simulink model "AutonomousScan"  (R2019a)
settings: Solver=FixedStepAuto  StartTime=0.0  StopTime=inf  FixedStep=0.001  RelTol=1e-3
libraries: dspnetwork x24, simulink_extras x3, etargetslib x1, dspmtrx3 x1, dspstat3 x1, simulink x1
(part 2 of 2)

== matlab function AutonomousScan/Trajectory Generation1 ==
  settings: updateMethod=DISCRETE
  data: pos_des output; current_pos input; record_data output; measured_force input; bias_good input
function [pos_des, record_data] = fcn( current_pos, measured_force, bias_good)
persistent k contact_made pnt 

if isempty(k)
    k = 1;
end

if isempty(contact_made)
    contact_made = false;
end

if isempty(pnt)
    pnt = 1;
end

%constants
trajectory = [0.45 0 0;
    0.475 -0.025 0;
    0.425 -0.025 0;
    0.415 0 0;
    0.485 0 0;
    0.475 0.025 0;
    0.425 0.025 0
    0.425 0.025 0];
pos_max_error = 0.0007;
pos_max_error_fine = 0.00005;
contact_force = -1.1;
smooth_traj = repmat(trajectory(1,:), 8000, 1);

%set contact flag by measuring z force
if bias_good == true && measured_force(3) <= contact_force
    contact_made = true;
end

%selective recording
if contact_made == true && mod(k,2) == 0
    record_data = 1;
else
    record_data = 0;
end

%generates vector between current and next point
vect = trajectory(k+1,:) - trajectory(k,:);

%generates trajectory between adjecent points
if contact_made == true
    for t = 1:5000
        smooth_traj(t,:) = trajectory(k,:) + (t/5000).*vect;
    end
    
    %SEND MORE OF FINAL POINT
    v = smooth_traj(5000,:);
    smooth_traj = [smooth_traj(1:5000,:); repmat(v,3000,1)];
    
    %SEND MORE OF EACH POINT
    %smooth_traj = repelem(smooth_traj(1:40,:), 1000, 1);
end

%send desired coordinates to robot
pos_des = smooth_traj(pnt, :).';

%checks if vector end point has been reached
err_pos = sum(abs(current_pos(1:2,1) - trajectory(k+1,1:2).'));
if contact_made == true && err_pos <= pos_max_error
    
    %switches to next set of adjacent points
    k = k + 1;
    
    %checks if end of trajectory
    if k == size(trajectory, 1)
        k = 7;
    end
    
    %reset counter
    pnt = 1;
end

if contact_made == true
    pnt = pnt + 1;
    if pnt == 8001
        pnt = 1;
    end
end

end


% %WAIT UNTIL REACHES EACH POINT
% err_pos_fine = sum(abs(current_pos(1:2,1) - desired_pos(1:2,1)));
% 
% pos_des = smooth_traj(pnt, :).';
% 
% if contact_made == true && err_pos_fine <= pos_max_error_fine
%     pnt = pnt +1;
%     if pnt == 8
%         pnt = 1;
%     end
% end

== matlab function AutonomousScan/MATLAB Function9 ==
  data: u input; V_cart_2 output; panda_pos input
function V_cart_2 = fcn(u, panda_pos)
persistent n
if isempty(n)
    n=1;
end

desPos = u(1:2,1)/100;

V_cart_2 = [desPos - panda_pos(1:2);0];

== matlab function AutonomousScan/MATLAB Function10 ==
  data: sensor input; y output
function y = fcn(sensor)
persistent n origSensor

if isempty(n)
    n = 1;
end

if isempty(origSensor)
    origSensor = zeros(7,1);
end

if n == 1 && sensor(1)~=0
    origSensor = sensor;
    
    n = 2;
end    

y = origSensor;

== matlab function AutonomousScan/MATLAB Function11 ==
  data: panda_pos input; y output; intraop input
function y = fcn(panda_pos, intraop)
persistent n origPanda

if isempty(n)
    n = 1;
end

if isempty(origPanda)
    origPanda = zeros(3,1);
end

if n == 1 && panda_pos(1)~=0 && intraop == 1
    origPanda = panda_pos;
    
    n = 2;
end    

y = origPanda;

== matlab function AutonomousScan/MATLAB Function12 ==
  data: y output; limit output
function [y, limit] = fcn()
persistent n

if isempty(n)
    n = 0;
end

n=n+1;

if n<=5000
    y = [0 0 0 0 0 0 0];
elseif n>5000 && n<= 10000
    y = [0 0 0 0 1 0 0];
elseif n>10000 && n<=15000
    y = [0 0 0 0 0 0 0];
else
    y = [0 0 0 0 1 0 0];
end


limit = n;

== matlab function AutonomousScan/MATLAB Function13 ==
  data: u input; y output
function y = fcn(u)
    for i = 1:3
        if u(i)>pi
            u(i) = u(i)-(2*pi)
        elseif u(i)<-pi
            u(i) = u(i)+(2*pi)
        end
    end
y = u;

== matlab function AutonomousScan/MATLAB Function14 ==
  data: rcm input; rotmat output; tip input; currentZ input
function rotmat = fcn(rcm, tip, currentZ)

newZ = tip-rcm;
newZ = newZ/norm(newZ);
normPlane = cross(currentZ, newZ);

axisRot = normPlane/norm(normPlane);
nx = axisRot(1);
ny = axisRot(2);
nz = axisRot(3);

theta = acos(dot(currentZ,newZ)/(norm(currentZ)*norm(newZ)));

v=1-cos(theta);
c=cos(theta);
s=sin(theta);

rotmat =[nx^2*v+c,nx*ny*v-nz*s,nx*nz*v+ny*s;...
                              nx*ny*v+nz*s,ny^2*v+c,ny*nz*v-nx*s;
                              nx*nz*v-ny*s,ny*nz*v+nx*s,nz^2*v+c];

== matlab function AutonomousScan/in general3 ==
  data: grad output; brad output; arad output; R input
function [grad,brad,arad] = so3_to_rpy(R)
sy = sqrt(R(3,2)^2 + R(3,3)^2);
if sy > eps
    % non singular
    grad = atan2(R(3,2),R(3,3));
    brad = atan2(-R(3,1),sy);
    arad = atan2(R(2,1),R(1,1));
else
    % singular
    grad = atan2(-R(2,3),R(2,2));
    brad = atan2(-R(3,1),sy);
    arad = 0;
end
end

== matlab function AutonomousScan/MATLAB Function15 ==
  data: R output; arad input; brad input; grad input
function R  = rot(arad,brad,grad)
%#codegen
Rz = [cos(arad) -sin(arad) 0; sin(arad) cos(arad) 0; 0 0 1];
Ry = [cos(brad) 0 sin(brad); 0 1 0; -sin(brad) 0 cos(brad)];
Rx = [1 0 0; 0 cos(grad) -sin(grad); 0 sin(grad) cos(grad)];
R = Rz * Ry * Rx;

== matlab function AutonomousScan/MATLAB Function16 ==
  data: R output; arad input; brad input; grad input
function R  = rot(arad,brad,grad)
%#codegen
Rz = [cos(arad) -sin(arad) 0; sin(arad) cos(arad) 0; 0 0 1];
Ry = [cos(brad) 0 sin(brad); 0 1 0; -sin(brad) 0 cos(brad)];
Rx = [1 0 0; 0 cos(grad) -sin(grad); 0 sin(grad) cos(grad)];
R = Rz * Ry * Rx;

== matlab function AutonomousScan/MATLAB Function18 ==
  data: R output; arad input; brad input; grad input
function R  = rot(arad,brad,grad)
%#codegen
Rz = [cos(arad) -sin(arad) 0; sin(arad) cos(arad) 0; 0 0 1];
Ry = [cos(brad) 0 sin(brad); 0 1 0; -sin(brad) 0 cos(brad)];
Rx = [1 0 0; 0 cos(grad) -sin(grad); 0 sin(grad) cos(grad)];
R = Rz * Ry * Rx;

== matlab function AutonomousScan/in general4 ==
  data: grad output; brad output; arad output; R input
function [grad,brad,arad] = so3_to_rpy(R)
sy = sqrt(R(3,2)^2 + R(3,3)^2);
if sy > eps
    % non singular
    grad = atan2(R(3,2),R(3,3));
    brad = atan2(-R(3,1),sy);
    arad = atan2(R(2,1),R(1,1));
else
    % singular
    grad = atan2(-R(2,3),R(2,2));
    brad = atan2(-R(3,1),sy);
    arad = 0;
end
end

== matlab function AutonomousScan/MATLAB Function20 ==
  data: u input; y output
function y = fcn(u)
    for i = 1:3
        if u(i)>pi
            u(i) = u(i)-(2*pi)
        elseif u(i)<-pi
            u(i) = u(i)+(2*pi)
        end
    end
y = u;

== matlab function AutonomousScan/MATLAB Function21 ==
  data: R input; T output; P input
function T = fcn(R, P)

T = [R P; 0 0 0 1];

== matlab function AutonomousScan/MATLAB Function22 ==
  data: u input; y output
function y = fcn(u)
y = u(1:3,end);

== matlab function AutonomousScan/MATLAB Function23 ==
  data: u input; y output
function y = fcn(u)
y=inv(u);

== matlab function AutonomousScan/MATLAB Function24 ==
  data: u input; y output
function y = fcn(u)
y=inv(u);

== matlab function AutonomousScan/MATLAB Function25 ==
  data: u input; y output
function y = fcn(u)
y = u(1:3,end);

== matlab function AutonomousScan/MATLAB Function26 ==
  data: pandaDes output; sensor input; quat output; sensorCurrent output; pandaCurrent input; rotZ input
function [pandaDes, quat, sensorCurrent]  = fcn(sensor, pandaCurrent, rotZ)
persistent transform transform2

if isempty(transform)
%     transform = [
%     0.0157   -0.0208   -0.9820   -0.0000
%     1.0071    0.0053    0.0197    0.0000
%     0.0034   -1.0071    0.0285   -0.0000
%     0.4598   -0.2811    0.0175    1.0000];

transform = [
    0.1742    0.9918    0.5463    0.0000
    0.8595   -0.7297   -0.0298    0.0000
   -0.1544   -0.9591   -0.0756   -0.0000
    0.3959   -0.3642    0.3008    1.0000
];
end


if isempty(transform2)
    transform2 = [
    0.0157   -0.0208   -0.9820   -0.0000
    1.0071    0.0053    0.0197    0.0000
    0.0034   -1.0071    0.0285   -0.0000
    0.4598   -0.2811    0.0175    1.0000];

end

sensorPos = [sensor(1:3)'./1000 1];
pandaPos = sensorPos * transform;
sensorCurrent = sensorPos*transform2;

% pandaPos(1) = pandaPos(1) - 0.2*sin(rotZ) + 0.0036;
% pandaPos(2) = pandaPos(2) - 0.2*cos(rotZ) - 0.0092;
%pandaPos(1) = sensorCurrent(1)-(abs(pandaPos(1)-sensorCurrent(1)))*sin(rotZ);
%pandaPos(2) = sensorCurrent(2)-(abs(pandaPos(2)-sensorCurrent(2)))*cos(rotZ);


if abs(sensorPos(1)) > 1000 || abs(sensorPos(2)) > 1000 || abs(sensorPos(3)) > 1000
    pandaPos = [pandaCurrent(1) pandaCurrent(2) pandaCurrent(3) 1];
end

pandaDes = [pandaPos(1:2) 0]';


quat = sensor(4:7);

== matlab function AutonomousScan/MATLAB Function27 ==
  data: u input; y output
function y = fcn(u)
    for i = 1:3
        if u(i)>pi
            u(i) = u(i)-(2*pi)
        elseif u(i)<-pi
            u(i) = u(i)+(2*pi)
        end
    end
y = u;

== matlab function AutonomousScan/Trajectory Generation (works) ==
  settings: updateMethod=DISCRETE
  data: shutter_fb input; pos_des output; current_pos input; record_data output; measured_force input; bias_good input; shutter output; pnts output; scan_complete output
function [pos_des, record_data, shutter, pnts, scan_complete] = fcn(shutter_fb, current_pos, measured_force, bias_good)
persistent k contact_made pnt shutter_pass

if isempty(k)
    k = 1;
end

if isempty(contact_made)
    contact_made = false;
end

if isempty(pnt)
    pnt = 1;
end

if isempty(shutter_pass)
    shutter_pass = 0;
end

%change to 0 when need to scan
scan_complete = 1;

%constants
trajectory = [0.45 0 0;
    0.475 -0.025 0;
    0.425 -0.025 0;
    0.415 0 0;
    0.485 0 0;
    0.475 0.025 0;
    0.425 0.025 0
    0.425 0.025 0];
pos_max_error_fine = 0.0001;
x_dist = 0.00125; %(0.475-0.425)/25
contact_force = -1.1;
% num_points = ceil(abs(trajectory(k+1,1)-trajectory(k,1))/x_dist);
num_points = ceil(abs(max(trajectory(:,1))-min(trajectory(:,1)))/x_dist)+1;

smooth_traj = repmat(trajectory(1,:), num_points, 1); 
shutter = 0;

%set contact flag by measuring z force
if bias_good == true && measured_force(3) <= contact_force
    contact_made = true;
end

%selective recording
% if contact_made == true && mod(k,2) == 0
if mod(k,2) == 0
    record_data = 1;
else
    record_data = 0;
end

%generates trajectory between adjecent points
if record_data == 1
    if trajectory(k,1) > trajectory(k+1,1)
        x_dist = -x_dist;
    end
        
    for t = 1:num_points
        smooth_traj(t,:) = [trajectory(k,1)+(t-1)*x_dist trajectory(k,2) trajectory(k,3)]; 
    end

elseif contact_made == true && record_data == 0 
    for t = 1:num_points
        smooth_traj(t,:) = trajectory(k+1,:);
    end
end

%send desired coordinates to robot
pos_des = smooth_traj(pnt, :).';

err_pos_fine = sum(abs(current_pos(1:2,1) - pos_des(1:2,1)));
if record_data == 1 && err_pos_fine <= pos_max_error_fine

    shutter_pass = 1; 
    
    if shutter_fb == 1
        pnt = pnt + 1;
        if pnt > num_points
            pnt = 1;
        end
        shutter_pass = 0;
    end
end

%checks if vector end point has been reached
err_pos = sum(abs(current_pos(1:2,1) - trajectory(k+1,1:2).'));
if contact_made == true && err_pos <= pos_max_error_fine
    
    shutter_pass = 1;
    
    if shutter_fb == 1
        %switches to next set of adjacent points
        k = k + 1;
        
        %checks if end of trajectory
        if k == size(trajectory, 1)
            k = size(trajectory, 1) - 1;
        end
        scan_complete = 1;
        %reset counter
        pnt = 1;
        shutter_pass = 0;
    end
    
    if k == size(trajectory, 1) - 1
        shutter_pass = 0;
    end
end

if shutter_pass == 1 && shutter_fb ~= 1
    shutter = 1;
end



pnts = pnt;
end

== matlab function AutonomousScan/MATLAB Function28 ==
  data: pandaPos input; pandaDes output
function pandaDes   = safetybox(pandaPos)
safetyboxX = [0.1 0.55];
safetyboxY = [-0.25 0.18];

if pandaPos(1) < safetyboxX(1)
    pandaPos(1) = safetyboxX(1);
elseif pandaPos(1) > safetyboxX(2)
    pandaPos(1) = safetyboxX(2);
end

if pandaPos(2) < safetyboxY(1)
    pandaPos(2) = safetyboxY(1);
elseif pandaPos(2) > safetyboxY(2)
    pandaPos(2) = safetyboxY(2);
end

pandaDes = [pandaPos(1:2); 0];

== matlab function AutonomousScan/MATLAB Function29 ==
  data: motoman_transform output; message input; hole output
function [motoman_transform, hole] = transform(message)

motoman_transform = [message(4:6)' ,message(1); message(7:9)', message(2); message(10:12)', message(3); 0 0 0 1];

current_motoman = [
    0.07043 0.9957 -0.06055 0.4181; 
    -0.02056 0.06214 0.9979 -0.06345; 
    0.9973 -0.06903 0.02485 0.2356]; 

newrotm = motoman_transform(1:3,1:3)*current_motoman(1:3,1:3); 

%motoman_offset = [1 0 0 (0.08352*sin(message(15)+2.8798)); 0 1 0 (0.08352*cos(message(15)+2.8798)); 0 0 1 -0.03; 0 0 0 1];
motoman_offset = [1 0 0 0.08352; 0 1 0 0.0108; 0 0 1 -0.03; 0 0 0 1];

desired_pos = newrotm*motoman_offset(1:3,4) + current_motoman(1:3,4);

transform = [
    0.0004   -0.9408    0.0079    0.0000
    0.9961    0.0739    0.0126   -0.0000
    0.0018   -0.0364    1.0297   -0.0000
    0.4523    0.5418   -0.1090    1.0000
];

tf = transform'*[motoman_transform(1:3,1:3) desired_pos; 0 0 0 1]; 
%tf = transform' *motoman_offset * motoman_transform  ; 

hole = tf(1:3,4);
end

== matlab function AutonomousScan/in general1 ==
  data: grad output; brad output; arad output; R input
function [grad,brad,arad] = so3_to_rpy(R)
sy = sqrt(R(3,2)^2 + R(3,3)^2);
if sy > eps
    % non singular
    grad = atan2(R(3,2),R(3,3));
    brad = atan2(-R(3,1),sy);
    arad = atan2(R(2,1),R(1,1));
else
    % singular
    grad = atan2(-R(2,3),R(2,2));
    brad = atan2(-R(3,1),sy);
    arad = 0;
end
end

== matlab function AutonomousScan/MATLAB Function30 ==
  data: rotZ output; input input
function rotZ   = filter(input)
persistent rotZ_dummy

if isempty(rotZ_dummy)
    rotZ_dummy = 0;
end 

if input > 4
    rotZ = rotZ_dummy;
else
    rotZ_dummy = input;
    rotZ = input;
end  
    

end

== matlab function AutonomousScan/MATLAB Function31 ==
  data: needletip_pos output; hole input; sensor input; needle output; unitneedle output
function [needletip_pos, needle, unitneedle]  = offset(hole, sensor)
persistent needletip_dummy

if isempty(needletip_dummy)
    needletip_dummy = [0.5 0 0];
end 

needle = [(hole(1) - sensor(1)) (hole(2) - sensor(2)) 0]; 

unitneedle = needle/norm(needle);  

needletip_test = [(sensor(1) + 0.2*unitneedle(1)) (sensor(2) + 0.2*unitneedle(2)) 0];

if abs(needletip_test(1)) > 1000 || abs(needletip_test(2)) > 1000
    needletip_pos = needletip_dummy;
else
    needletip_dummy = needletip_test;
    needletip_pos = needletip_test;
end  
    

end

== matlab function AutonomousScan/MATLAB Function32 ==
  data: motoman_transform output; message input; needletip_pos output; sensor input; motoman_pos output; motoman_rpy output
function [motoman_transform, needletip_pos, motoman_pos, motoman_rpy]  = transform(message, sensor)
persistent needletip_dummy

if isempty(needletip_dummy)
    needletip_dummy = [0.5 0 0];
end 

motoman_transform = [message(4:6)' ,message(1); message(7:9)', message(2); message(10:12)', message(3); 0 0 0 1];
%current_motoman = [0.0153 0.0582 0.9982 0.4147; -0.0478 -0.9971 0.0589 0.0060; 0.9987 -0.0486 -0.0125 0.2397]; 
%newrotm = motoman_transform(1:3,1:3)*current_motoman(1:3,1:3); 
%motoman_offset = [1 0 0 (0.08352*sin(message(15)+2.8798)); 0 1 0 (0.08352*cos(message(15)+2.8798)); 0 0 1 -0.03; 0 0 0 1];
%motoman_offset = [1 0 0 0.08352; 0 1 0 0.0108; 0 0 1 -0.03; 0 0 0 1];

current_motoman = [
    0.07043 0.9957 -0.06055 0.4181; 
    -0.02056 0.06214 0.9979 -0.06345; 
    0.9973 -0.06903 0.02485 0.2356]; 

transform_sensor = [
    0.0157   -0.0208   -0.9820   -0.0000
    1.0071    0.0053    0.0197    0.0000
    0.0034   -1.0071    0.0285   -0.0000
    0.4598   -0.2811    0.0175    1.0000];

transform_motoman = [    
    0.0004   -0.9408    0.0079    0.0000
    0.9961    0.0739    0.0126   -0.0000
    0.0018   -0.0364    1.0297   -0.0000
    0.4523    0.5418   -0.1090    1.0000];

%Motoman position in panda base frame and motoman euler angles
motoman_pos = motoman_transform(1:4,4)' * transform_motoman; 
motoman_rpy = message(13:15); 

%Three points on the needle guide in sensor frame
needleguideA = [-0.1179 0.0185 -0.4357 1];
needleguideB = [-0.1804 0.019 -0.4274 1];
needleguideC = [-0.1172 -0.0366 -0.4349 1];

%Transform needle guide points from sensor frame to panda base frame
a_tf_p = needleguideA * transform_sensor;
b_tf_p = needleguideB * transform_sensor; 
c_tf_p = needleguideC * transform_sensor;

%Transform needle guide points from panda base frame to motoman base frame
a_tf_m = a_tf_p / transform_motoman;
b_tf_m = b_tf_p / transform_motoman;
c_tf_m = c_tf_p / transform_motoman;

%Calculating the position of all three points in the new motoman position
a_rot_m = motoman_transform(1:3,1:3) / current_motoman(1:3,1:3) * a_tf_m(1:3)';
b_rot_m = motoman_transform(1:3,1:3) / current_motoman(1:3,1:3) * b_tf_m(1:3)';
c_rot_m = motoman_transform(1:3,1:3) / current_motoman(1:3,1:3) * c_tf_m(1:3)';

%Transform rotated points back to panda base frame
a_rot_p = [a_rot_m; 1]' * transform_motoman; 
b_rot_p = [b_rot_m; 1]' * transform_motoman;
c_rot_p = [c_rot_m; 1]' * transform_motoman;

%Create two vectors about point a so they are in the same plane as the
%needle guide
ng_ab = b_rot_p - a_rot_p; 
ng_ac = c_rot_p - a_rot_p; 

%Calculating the normal vector to the plane of the needle guide
normvect_p = cross(ng_ab(1:3), ng_ac(1:3));

%Calculating the unit vector of the normal vector
unitnormvect_p = normvect_p(1:3)/norm(normvect_p(1:3));

%Add 20 cm from the location of the sensor in the direction of the unit
%vector to get to the needle tip
needletip_test = [(sensor(1) + 0.2*unitnormvect_p(1)) (sensor(2) + 0.2*unitnormvect_p(2)) 0];

%Check if the calculated needle tip position is acceptable
if abs(needletip_test(1)) > 1000 || abs(needletip_test(2)) > 1000
    needletip_pos = needletip_dummy;
else
    needletip_dummy = needletip_test;
    needletip_pos = needletip_test;
end  


%tf = transform'*[motoman_transform(1:3,1:3) desired_pos; 0 0 0 1]; 
%tf = transform' *motoman_offset * motoman_transform  ; 
%hole = tf(1:3,4);
end

== matlab function AutonomousScan/MATLAB Function34 ==
  data: u input; y output
function y = fcn(u)
    for i = 1:3
        if u(i)>pi
            u(i) = u(i)-(2*pi)
        elseif u(i)<-pi
            u(i) = u(i)+(2*pi)
        end
    end
y = u;

== matlab function AutonomousScan/MATLAB Function19 ==
  data: R_err output; R_des input; R_i input
function R_err  = R_err(R_des,R_i)
%#codegen
R_err = R_des*R_i';

== matlab function AutonomousScan/MATLAB Function33 ==
  data: u input; stop output
function stop = fcn(u)
if u(16) == 1 && u(17) == 1
    stop = 1;
else
    stop = 0;
end

== matlab function AutonomousScan/MATLAB Function17 ==
  data: u input; y output
function y = fcn(u)

y = u(:,3);
